simulink model "gm_sampleModel1853_3_sub_sub_sub"  (R2023a)
settings: Solver=VariableStepAuto  StartTime=0.0  StopTime=10.0  RelTol=1e-3
libraries: hdlsllib x5, simulink x3
settings Model: Creator=user1  LastModifiedBy=user1
settings OptimizationCC: BlockReduction=off  ConditionallyExecuteInputs=off
settings DebuggingCC: InheritedTsInSrcMsg=none

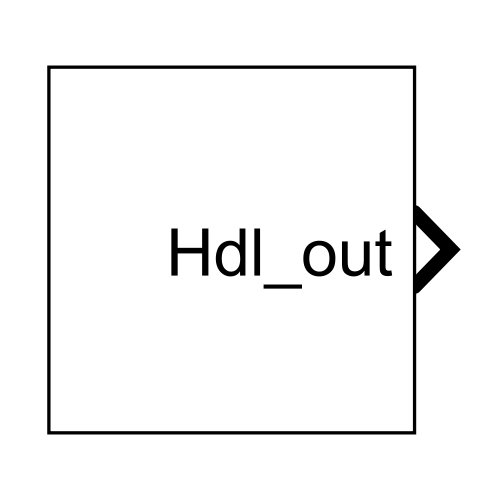
[thumbnail: Simulink's stored preview of the top-level diagram]
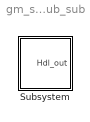
== system gm_sampleModel1853_3_sub_sub_sub ==
  Subsystem : Subsystem

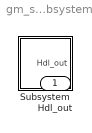
== system gm_sampleModel1853_3_sub_sub_sub/Subsystem ==
  Subsystem : Subsystem
  Hdl_out : Outport  OutDataTypeStr=uint8

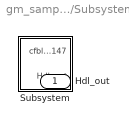
== system gm_sampleModel1853_3_sub_sub_sub/Subsystem/Subsystem ==
  Subsystem : Subsystem
  Hdl_out : Outport  OutDataTypeStr=uint8

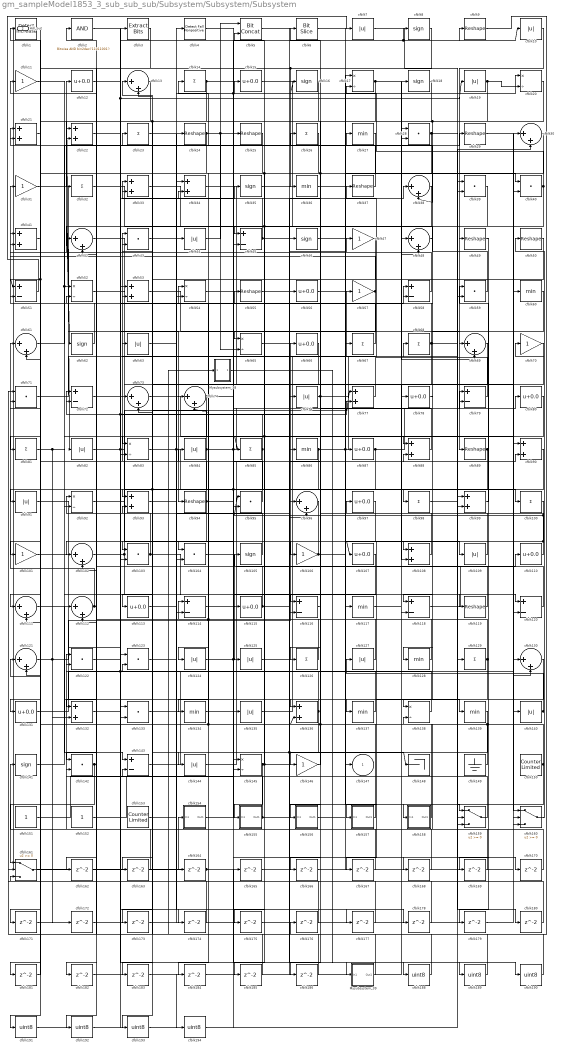
== system gm_sampleModel1853_3_sub_sub_sub/Subsystem/Subsystem/Subsystem ==
  Mysubsystem_38 : Subsystem  TreatAsAtomicUnit=on  RTWFcnName=Mysubsystem_38
      settings: RTWFcnNameOpts=User specified  RTWFileNameOpts=Use function name
  Mysubsystem_39 : Subsystem  TreatAsAtomicUnit=on  RTWFcnName=Mysubsystem_39
      settings: RTWFcnNameOpts=User specified  RTWFileNameOpts=Use function name
  cfblk1 : simulink/Logic and Bit Operations/Detect Increase  vinit=0.0  OutDataTypeStr=uint8
      settings: LibrarySourceBlock=|
      | hdlsllib/Logic and Bit
      | Operations/Detect
      | Increase
  cfblk{7,10,19,44,63,76,82,84,91,109,124..125,127,135,140,144} (16 alike) : Abs  OutDataTypeStr=uint8  SaturateOnIntegerOverflow=off
  cfblk{14,23,26,32,67..68,81,85,98,100,126,129} (12 alike) : Sum  Inputs=+  OutDataTypeStr=uint8
  cfblk{11,31,47,57,70,101,106,146} (8 alike) : Gain  OutDataTypeStr=uint8
  cfblk{13,30,38,42,48,61,69,73..74,96,102,111..112,121,130} (15 alike) : Sum  Inputs=|++  OutDataTypeStr=uint8
  cfblk{28,39..40,43,59,71,95,103..104,122..123,133,142} (13 alike) : DotProduct  OutDataTypeStr=uint8
  cfblk{8,16,18,35,46,62,105,141} (8 alike) : Signum
  cfblk{12,15,56,66,78,80,87,97,107,110,113,115,131} (13 alike) : Bias  Bias=0.0  SaturateOnIntegerOverflow=off
  cfblk{21..22,33..34,41,53,77,88,90,93,99,108,132,136} (14 alike) : Sum  OutDataTypeStr=uint8
  cfblk{45,51,58,72,79,114,116,118,120,143} (10 alike) : Sum  Inputs=+-  OutDataTypeStr=uint8
  cfblk{27,36,60,86,117,128,134,137,139} (9 alike) : MinMax  OutDataTypeStr=uint8
  cfblk{9,24..25,29,37,49..50,55,89,94,119} (11 alike) : Reshape
  cfblk{17,20,52,54,65,83,92,138,145} (9 alike) : Product  Inputs=*/  OutDataTypeStr=uint8  RndMeth=Zero  SaturateOnIntegerOverflow=on
  cfblk148 : Terminator
  cfblk149 : Ground
  cfblk150 : hdlsllib/Sources/Counter Limited  uplimit=7  tsamp=-1
  cfblk151 : Constant  OutDataTypeStr=uint8  SampleTime=-1
  cfblk152 : Constant  OutDataTypeStr=uint8  SampleTime=-1
  cfblk153 : hdlsllib/Sources/Counter Limited  uplimit=7  tsamp=-1
  cfblk154 : Subsystem
      settings: LibrarySourceBlock=|
      | hdlsllib/Ports &
      | Subsystems/Subsystem
  cfblk155 : Subsystem
      settings: LibrarySourceBlock=|
      | hdlsllib/Ports &
      | Subsystems/Subsystem
  cfblk156 : Subsystem
      settings: LibrarySourceBlock=|
      | hdlsllib/Ports &
      | Subsystems/Subsystem
  cfblk157 : Subsystem
      settings: LibrarySourceBlock=|
      | hdlsllib/Ports &
      | Subsystems/Subsystem
  cfblk158 : Subsystem
      settings: LibrarySourceBlock=|
      | hdlsllib/Ports &
      | Subsystems/Subsystem
  cfblk159 : Switch  OutDataTypeStr=uint8  SaturateOnIntegerOverflow=off  InputSameDT=off
  cfblk160 : Switch  OutDataTypeStr=uint8  SaturateOnIntegerOverflow=off  InputSameDT=off
  cfblk161 : Switch  OutDataTypeStr=uint8  SaturateOnIntegerOverflow=off  InputSameDT=off
  cfblk{162..186} (25 alike) : Delay  SampleTime=1
  cfblk{188..194} (7 alike) : DataTypeConversion  OutDataTypeStr=uint8  SaturateOnIntegerOverflow=off  RndMeth=Floor
  cfblk2 : simulink/Logic and Bit Operations/Bitwise Operator  logicop=AND  UseBitMask=on  BitMask=bin2dec('11011001')  BitMaskRealWorld=Stored Integer
      settings: LibrarySourceBlock=|
      | hdlsllib/Logic and Bit
      | Operations/Bitwise
      | Operator
  cfblk3 : simulink/Logic and Bit Operations/Extract Bits  bitsToExtract=Upper half  numBits=8  bitIdxRange=[0 7]  outScalingMode=Preserve fixed-point scaling
      settings: LibrarySourceBlock=|
      | hdlsllib/Logic and Bit
      | Operations/Extract Bits
  cfblk4 : hdlsllib/Logic and Bit Operations/Detect Fall Nonpositive  vinit=0  OutDataTypeStr=uint8
  cfblk5 : hdlsllib/Logic and Bit Operations/Bit Concat  numInputs=2
  cfblk6 : hdlsllib/Logic and Bit Operations/Bit Slice  lidx=7  ridx=0
  cfblk147 : Outport  OutDataTypeStr=uint8  VectorParamsAs1DForOutWhenUnconnected=off
  Hdl_out : Outport  Port=2  OutDataTypeStr=uint8
  wires:
  Mysubsystem_39/1(Out1) -> Mysubsystem_38/1(In1)
  Mysubsystem_38/1(Out1) -> Mysubsystem_39/1(In1)
  cfblk194/1 -> cfblk39/2
  cfblk183/1 -> cfblk194/1
  cfblk193/1 -> cfblk39/1
  cfblk192/1 -> cfblk123/1
  cfblk39/1 -> cfblk192/1
  cfblk191/1 -> cfblk165/1
  cfblk13/1 -> cfblk191/1
  cfblk190/1 -> cfblk123/2
  cfblk165/1 -> cfblk190/1
  cfblk189/1 -> cfblk71/1
  cfblk2/1 -> cfblk189/1
  cfblk188/1 -> cfblk2/1
  cfblk186/1 -> cfblk161/3
  cfblk185/1 -> cfblk102/2
  cfblk184/1 -> cfblk48/1
  cfblk70/1 -> cfblk184/1
  cfblk182/1 -> cfblk96/2
  cfblk181/1 -> cfblk61/2
  cfblk21/1 -> cfblk181/1
  cfblk180/1 -> cfblk161/2
  cfblk179/1 -> cfblk40/2
  cfblk90/1 -> cfblk179/1
  cfblk178/1 -> cfblk143/2
  cfblk63/1 -> cfblk178/1
  cfblk177/1 -> cfblk33/2
  cfblk176/1 -> cfblk112/2
  cfblk9/1 -> cfblk176/1
  cfblk175/1 -> cfblk118/2
  cfblk174/1 -> cfblk53/1
  cfblk12/1 -> cfblk174/1
  cfblk173/1 -> cfblk28/2
  cfblk172/1 -> cfblk34/1
  cfblk171/1 -> cfblk160/3
  cfblk170/1 -> cfblk138/2
  cfblk4/1 -> cfblk170/1
  cfblk169/1 -> cfblk121/1
  cfblk168/1 -> cfblk73/2
  cfblk35/1 -> cfblk168/1
  cfblk167/1 -> cfblk111/2
  cfblk100/1 -> cfblk167/1
  cfblk166/1 -> cfblk130/2
  cfblk164/1 -> cfblk17/1, Hdl_out/1
  cfblk23/1 -> cfblk164/1
  cfblk163/1 -> cfblk142/2
  cfblk66/1 -> cfblk163/1
  cfblk162/1 -> cfblk160/2
  cfblk43/1 -> cfblk27/1
  cfblk53/1 -> cfblk69/1
  cfblk108/1 -> cfblk97/1
  cfblk114/1 -> cfblk78/1
  cfblk122/1 -> cfblk58/2, cfblk77/1
  cfblk154/1(Out1) -> cfblk8/1, cfblk10/1, cfblk16/1
  cfblk94/1 -> cfblk25/1, cfblk103/2, cfblk51/2
  cfblk106/1 -> cfblk102/1, cfblk159/3
  cfblk107/1 -> cfblk145/2
  cfblk71/1 -> cfblk46/1
  cfblk98/1 -> cfblk30/2
  cfblk160/1 -> cfblk50/1
  cfblk111/1 -> cfblk143/1
  cfblk65/1 -> cfblk99/2
  cfblk158/1(Out1) -> cfblk55/1
  cfblk113/1 -> cfblk4/1
  cfblk85/1 -> cfblk142/1, cfblk95/2, cfblk72/1
  cfblk24/1 -> cfblk65/2, cfblk188/1, cfblk54/2
  cfblk45/1 -> cfblk34/2, cfblk158/1(In1)
  cfblk81/1 -> cfblk136/1, cfblk172/1
  cfblk5/1 -> cfblk159/1, cfblk148/1
  cfblk32/1 -> cfblk147/1, cfblk87/1
  cfblk40/1 -> cfblk17/2, cfblk162/1
  cfblk125/1 -> cfblk68/1
  cfblk74/1 -> cfblk88/1, cfblk92/2
  cfblk150/1 -> cfblk5/2, cfblk116/2, cfblk159/2
  cfblk97/1 -> cfblk134/1
  cfblk22/1 -> cfblk19/1, cfblk9/1
  cfblk25/1 -> cfblk111/1, cfblk51/1
  cfblk134/1 -> cfblk20/1
  cfblk7/1 -> cfblk99/1
  cfblk30/1 -> cfblk81/1
  cfblk76/1 -> cfblk126/1, cfblk59/2
  cfblk37/1 -> cfblk14/1
  cfblk136/1 -> cfblk93/2, cfblk173/1
  cfblk6/1 -> cfblk119/1
  cfblk129/1 -> cfblk23/1, cfblk157/1(In1)
  cfblk11/1 -> cfblk52/1, cfblk114/2
  cfblk72/1 -> cfblk116/1
  cfblk86/1 -> cfblk48/2, cfblk104/2
  cfblk110/1 -> cfblk95/1, cfblk72/2, cfblk107/1
  cfblk152/1 -> cfblk45/2
  cfblk87/1 -> cfblk79/1, cfblk186/1
  cfblk139/1 -> cfblk136/2, cfblk193/1
  cfblk145/1 -> cfblk105/1, cfblk38/1, cfblk155/1(In1)
  cfblk109/1 -> cfblk33/1
  cfblk14/1 -> cfblk42/1, cfblk137/1
  cfblk61/1 -> cfblk29/1
  cfblk117/1 -> cfblk80/1
  cfblk155/1(Out1) -> cfblk43/2, cfblk177/1
  cfblk92/1 -> cfblk145/1
  cfblk146/1 -> cfblk86/1
  cfblk119/1 -> cfblk53/2
  cfblk103/1 -> cfblk135/1, cfblk42/2
  cfblk26/1 -> cfblk144/1
  cfblk36/1 -> cfblk40/1
  cfblk118/1 -> cfblk60/1
  cfblk55/1 -> cfblk47/1
  cfblk80/1 -> cfblk83/1
  cfblk46/1 -> cfblk67/1
  cfblk16/1 -> cfblk103/1, cfblk132/1
  cfblk104/1 -> cfblk125/1
  cfblk29/1 -> cfblk160/1
  cfblk47/1 -> cfblk93/1
  cfblk124/1 -> cfblk18/1, cfblk90/2
  cfblk105/1 -> cfblk63/1
  cfblk88/1 -> cfblk26/1
  cfblk137/1 -> cfblk122/2
  cfblk161/1 -> cfblk154/1(In1)
  cfblk77/1 -> cfblk13/2
  cfblk102/1 -> cfblk76/1, cfblk120/1
  cfblk60/1 -> cfblk128/1
  cfblk27/1 -> cfblk65/1, cfblk166/1
  cfblk28/1 -> cfblk121/2, cfblk185/1, cfblk120/2
  cfblk54/1 -> cfblk130/1
  cfblk138/1 -> cfblk6/1
  cfblk3/1 -> cfblk32/1
  cfblk59/1 -> cfblk22/1
  cfblk99/1 -> cfblk59/1
  cfblk149/1 -> cfblk71/2
  cfblk31/1 -> cfblk74/1
  cfblk8/1 -> cfblk36/1, cfblk131/1
  cfblk52/1 -> cfblk108/2
  cfblk62/1 -> cfblk41/2
  cfblk126/1 -> cfblk54/1
  cfblk123/1 -> cfblk96/1
  cfblk132/1 -> cfblk73/1
  cfblk156/1(Out1) -> cfblk117/1
  cfblk73/1 -> cfblk140/1
  cfblk144/1 -> cfblk110/1
  cfblk143/1 -> cfblk28/1
  cfblk48/1 -> cfblk118/1
  cfblk116/1 -> cfblk156/1(In1)
  cfblk157/1(Out1) -> cfblk13/1, cfblk74/2
  cfblk78/1 -> cfblk138/1
  cfblk18/1 -> cfblk133/2
  cfblk128/1 -> cfblk114/1
  cfblk79/1 -> cfblk37/1
  cfblk56/1 -> cfblk109/1
  cfblk131/1 -> cfblk3/1, cfblk90/1
  cfblk151/1 -> cfblk24/1
  cfblk141/1 -> cfblk112/1
  cfblk50/1 -> cfblk85/1, cfblk115/1
  cfblk120/1 -> cfblk41/1
  cfblk93/1 -> cfblk15/1
  cfblk140/1 -> cfblk127/1, cfblk70/1
  cfblk91/1 -> cfblk133/1
  cfblk133/1 -> cfblk30/1
  cfblk41/1 -> cfblk91/1
  cfblk127/1 -> cfblk84/1, cfblk21/1
  cfblk67/1 -> cfblk1/1
  cfblk142/1 -> cfblk161/1, cfblk52/2
  cfblk82/1 -> cfblk100/1, cfblk35/1
  cfblk115/1 -> cfblk11/1, cfblk88/2
  cfblk51/1 -> cfblk7/1
  cfblk38/1 -> cfblk62/1, cfblk175/1
  cfblk84/1 -> cfblk182/1, cfblk183/1, cfblk56/1, cfblk79/2, cfblk21/2
  cfblk96/1 -> cfblk106/1
  cfblk19/1 -> cfblk82/1, cfblk38/2, cfblk20/2
  cfblk33/1 -> cfblk45/1
  cfblk130/1 -> cfblk141/1
  cfblk83/1 -> cfblk98/1, cfblk77/2
  cfblk10/1 -> cfblk49/1
  cfblk1/1 -> cfblk101/1
  cfblk34/1 -> cfblk129/1
  cfblk44/1 -> cfblk5/1
  cfblk49/1 -> cfblk108/1
  cfblk159/1 -> cfblk122/1
  cfblk101/1 -> cfblk139/1
  cfblk135/1 -> cfblk57/1
  cfblk95/1 -> cfblk43/1
  cfblk89/1 -> cfblk113/1, cfblk171/1, cfblk169/1
  cfblk153/1 -> cfblk44/1
  cfblk17/1 -> cfblk146/1, cfblk69/2
  cfblk68/1 -> cfblk124/1, cfblk22/2, cfblk180/1
  cfblk15/1 -> cfblk58/1
  cfblk42/1 -> cfblk104/1
  cfblk69/1 -> cfblk94/1
  cfblk57/1 -> cfblk31/1, cfblk83/2
  cfblk20/1 -> cfblk89/1
  cfblk121/1 -> cfblk66/1, cfblk132/2
  cfblk58/1 -> cfblk12/1
  cfblk112/1 -> cfblk61/1, cfblk92/1

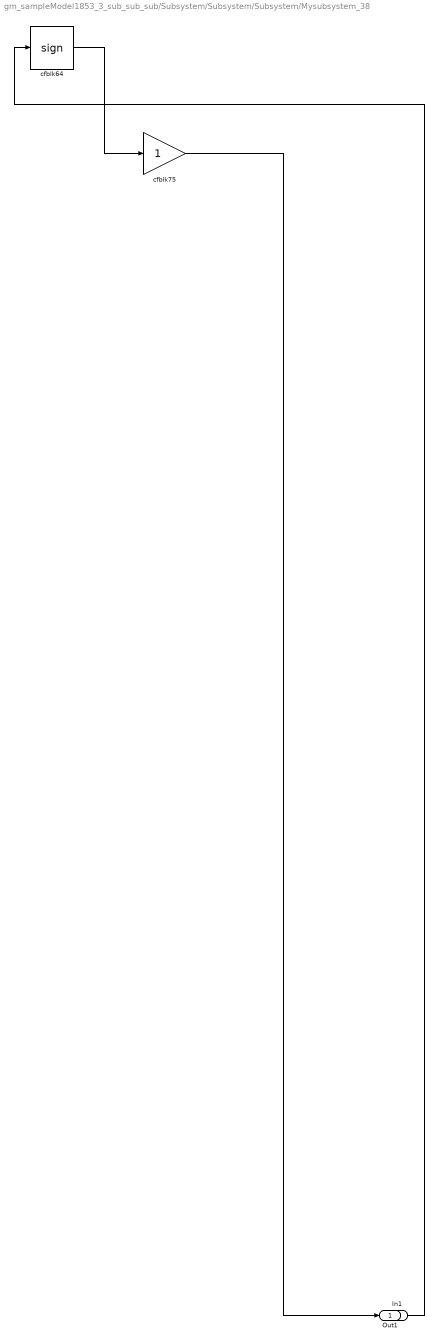
== system gm_sampleModel1853_3_sub_sub_sub/Subsystem/Subsystem/Subsystem/Mysubsystem_38 ==
  In1 : Inport
  cfblk64 : Signum
  cfblk75 : Gain
  Out1 : Outport
  wires:
  cfblk64/1 -> cfblk75/1
  cfblk75/1 -> Out1/1
  In1/1 -> cfblk64/1

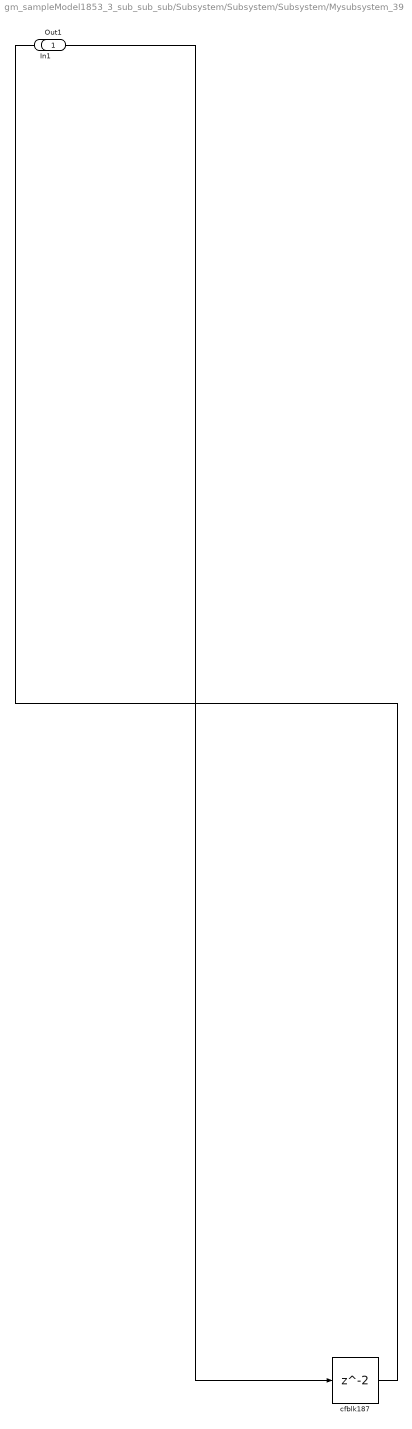
== system gm_sampleModel1853_3_sub_sub_sub/Subsystem/Subsystem/Subsystem/Mysubsystem_39 ==
  In1 : Inport
  cfblk187 : Delay  SampleTime=1
  Out1 : Outport
  wires:
  In1/1 -> cfblk187/1
  cfblk187/1 -> Out1/1

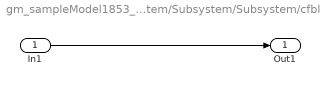
== system gm_sampleModel1853_3_sub_sub_sub/Subsystem/Subsystem/Subsystem/cfblk154 ==
  In1 : Inport
  Out1 : Outport
  wires:
  In1/1 -> Out1/1

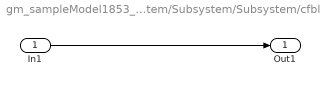
== system gm_sampleModel1853_3_sub_sub_sub/Subsystem/Subsystem/Subsystem/cfblk155 ==
  In1 : Inport
  Out1 : Outport
  wires:
  In1/1 -> Out1/1

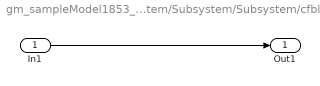
== system gm_sampleModel1853_3_sub_sub_sub/Subsystem/Subsystem/Subsystem/cfblk156 ==
  In1 : Inport
  Out1 : Outport
  wires:
  In1/1 -> Out1/1

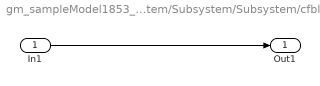
== system gm_sampleModel1853_3_sub_sub_sub/Subsystem/Subsystem/Subsystem/cfblk157 ==
  In1 : Inport
  Out1 : Outport
  wires:
  In1/1 -> Out1/1

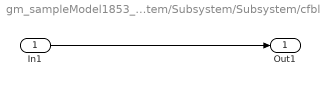
== system gm_sampleModel1853_3_sub_sub_sub/Subsystem/Subsystem/Subsystem/cfblk158 ==
  In1 : Inport
  Out1 : Outport
  wires:
  In1/1 -> Out1/1
